simulink model "dobbel_oppdatert_sim"  (R2023b)
settings: Solver=VariableStepAuto  StartTime=0.0  StopTime=inf  FixedStep=0.0001  RelTol=1e-6  AbsTol=1e-6
model workspace (MAT data in the model file):
  SL_ROS_VariableLengthArrays_MaxSizes.CommonInfo.ArrayTruncateAction = 'EmitWarning'
  SL_ROS_VariableLengthArrays_MaxSizes.MsgTypeMap = containers.Map
  SL_ROS_VariableLengthArrays_MaxSizes.MsgTypeMap.serialization.keys = {'std_msgs/Float64MultiArray'}
  SL_ROS_VariableLengthArrays_MaxSizes.MsgTypeMap.serialization.values{1}.PropertyName = 'data'
  SL_ROS_VariableLengthArrays_MaxSizes.MsgTypeMap.serialization.values{1}.DataType = 'double'
  SL_ROS_VariableLengthArrays_MaxSizes.MsgTypeMap.serialization.values{1}.MaxLength = 500
  SL_ROS_VariableLengthArrays_MaxSizes.MsgTypeMap.serialization.uniformity = 0
  SL_ROS_VariableLengthArrays_MaxSizes.MsgTypeMap.serialization.keyType = 'char'
  SL_ROS_VariableLengthArrays_MaxSizes.MsgTypeMap.serialization.valueType = 'any'
values from neighbouring files (symbols this model uses):
  B = 10    [LoneWolfParams.m]
  C = 1.9    [LoneWolfParams.m]
  D = 1    [LoneWolfParams.m]
  g = 9.81    [LoneWolfParams.m]
  Iz = (1/12) * m * (with^2 + len^2)    [LoneWolfParams.m]
  m = 375    [LoneWolfParams.m]
  xdotinit = 1e-3    (= 0.001)    [LoneWolfParams.m]
undefined symbols (not defined in the file or in its folder): latitude, longitude
libraries: ros2lib x11, simulink x2, dspstat3 x1, sldrtlib x1
settings Model: Creator=bakke  LastModifiedBy=lonewolf
settings SolverCC: AutoScaleAbsTol=off  EnableFixedStepZeroCrossing=on  MaxZcBracketingIterations=100
settings OptimizationCC: EnhancedBackFolding=on  PassReuseOutputArgsAs=Individual arguments  ZeroExternalMemoryAtStartup=off  ZeroInternalMemoryAtStartup=off  MaxStackSize=64  OptimizeBlockOrder=speed  DifferentSizesBufferReuse=on  OptimizationCustomize=off  EfficientTunableParamExpr=on
settings DebuggingCC: ParameterTunabilityLossMsg=error
settings HardwareCC: ProdBitPerLong=64  ProdHWDeviceType=Intel->x86-64 (Linux 64)  UseEmbeddedCoderFeatures=off
settings RTWCC: Description=Embedded Coder  SystemTargetFile=ert.tlc  HardwareBoard=Robot Operating System 2 (ROS 2)  TLCOptions="-aInlineSetEventsForThisBaseRateFcn=TLC_FALSE -aSuppressMultiTaskScheduler=TLC_FALSE  -aRateBasedStepFcn=0"  TemplateMakefile=ert_default_tmf  Toolchain=Colcon Tools  TargetLang=C++
settings CodeAppCC: ForceParamTrailComments=on  IgnoreCustomStorageClasses=off  OperatorAnnotations=on  SimulinkDataObjDesc=on  SFDataObjDesc=on  InsertBlockDesc=on
settings ERTTargetCC: CodeInterfacePackaging=C++ class  SupportNonInlinedSFcns=on  RootIOFormat=Structure reference

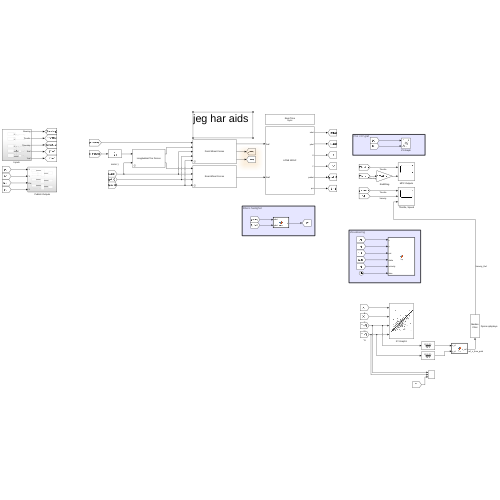
[thumbnail: Simulink's stored preview of the top-level diagram]
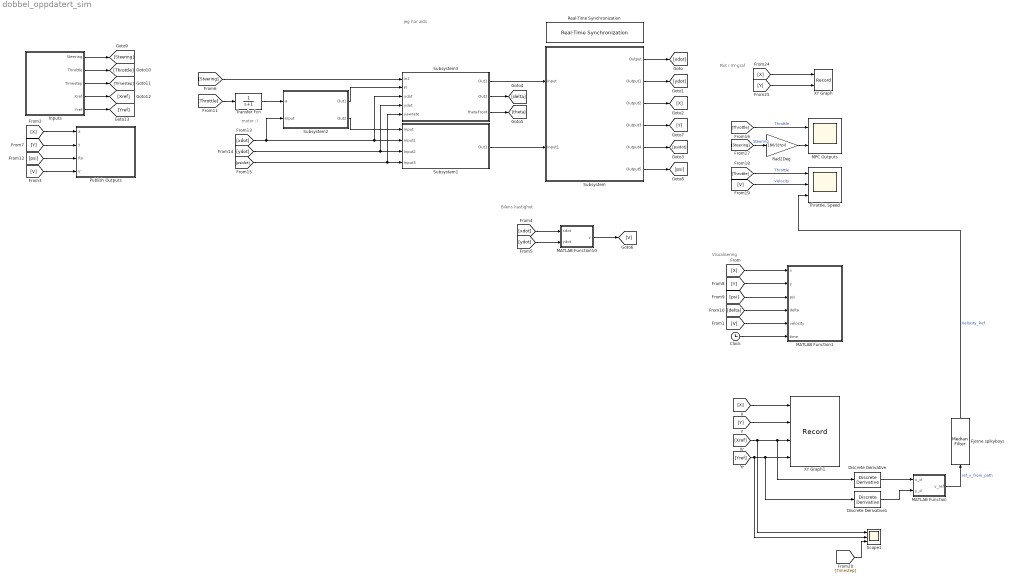
== system dobbel_oppdatert_sim ==
  note: motor :)
  note: jeg har aids
  note: Visualisering
  note: Plot i XY-graf
  note: Bilens hastighet
  Clock : Clock
  Discrete Derivative : simulink/Discrete/Discrete Derivative  gainval=1.0  ICPrevScaledInput=0.0  OutMin=[]  OutMax=[]  OutDataType=fixdt(1, 16)  OutScaling=2^-10  DoSatur=off
  Discrete Derivative1 : simulink/Discrete/Discrete Derivative  gainval=1.0  ICPrevScaledInput=0.0  OutMin=[]  OutMax=[]  OutDataType=fixdt(1, 16)  OutScaling=2^-10  DoSatur=off
  Fjerne spikyboys : dspstat3/Median Filter  WindowLength=5  SimulateUsing=Interpreted execution
      settings: LibrarySourceBlock=|
      | dspfdesign/Median
      | Filter
  Inputs : Subsystem
  MATLAB Function : MATLAB Function  TreatAsAtomicUnit=on
  MATLAB Function1 : MATLAB Function  TreatAsAtomicUnit=on
  MATLAB Function10 : MATLAB Function  TreatAsAtomicUnit=on
  MPC Outputs : Scope  NumInputPorts=2
  Publish Outputs : Subsystem
  Rad2Deg : Gain  Gain=180/(2*pi)
  Real-Time Synchronization : sldrtlib/Real-Time Synchronization  SampleTime=0.1  MaxMissedTicks=1000  ShowMissedTicks=off  YieldWhenWaiting=off
  Scope1 : Scope  NumInputPorts=3
  Subsystem : Subsystem
      mask Display: disp('LONE WOLF');
  Subsystem1 : Subsystem
      mask Display: disp('Rear Wheel Forces');
  Subsystem2 : Subsystem
      mask Display: disp('Longitudinal Tire Forces');
  Subsystem3 : Subsystem
      mask Display: disp('Front Wheel Forces');
  "Throttle, Speed" : Scope  NumInputPorts=3
  Transfer Fcn : TransferFcn  Denominator=[1 1]
  XY Graph : Record  FileSettingsInternal="{\"entries\":[{\"content\":{\"excelSettings\":{\"content\":{},\"type\":\"Streamout.ExcelSettings\"}},\"type\":\"Streamout.FileSettingStorage\",\"uuid\":\"\"}],\"packageUris\":[\"http:\\/\\/schema.mathworks.com\\/mf0\\/streamout_blocks\\/R2020a\"],\"version\":\"1.0\"}"  Layout=[1 1]  SignalsInternal="{\"entries\":[{\"content\":{\"signals\":[{\"content\":{\"blockPath\":[],\"dimensions\":[1],\"domain\":\"\",\"lineColor\":\"#d95319\",\"plots\":[ 1 ],\"port\":1,\"sid\":[\"\"],\"signalID\":1,\"signalName\":\"From24\"},\"type\":\"RecordBlkView.Signal\",\"uuid\":\"\"},{\"content\":{\"blockPath\":[],\"dimensions\":[1],\"domain\":\"\",\"lineColor\":\"#edb120\",\"plots\":[ 1 ],\"port\":2,\"sid\":[\"\"],\"signalID\":2,\"signalName\":\"From25\"},\"type\":\"RecordBlkView.Signal\",\"uuid\":\"\"}]},\"type\":\"RecordBlkView.InputSignals\",\"uuid\":\"\"}],\"packageUris\":[\"http:\\/\\/schema.mathworks.com\\/mf0\\/streamout_blocks\\/R2020a\"],\"version\":\"1.0\"}"  VisualizationBindings="{\"xyplotplugin\":{\"info\":[{\"series\":[{\"bindingParametersList\":[{\"parameter\":\"X-Axis\",\"signalID\":1,\"signalName\":\"From24\"},{\"parameter\":\"Y-Axis\",\"signalID\":2,\"signalName\":\"From25\"}],\"seriesID\":0}],\"subplotID\":1}]}}"  CompatibilityTag=XY
  XY Graph1 : Record  FileSettingsInternal="{\"entries\":[{\"content\":{\"excelSettings\":{\"content\":{},\"type\":\"Streamout.ExcelSettings\"}},\"type\":\"Streamout.FileSettingStorage\",\"uuid\":\"\"}],\"packageUris\":[\"http:\\/\\/schema.mathworks.com\\/mf0\\/streamout_blocks\\/R2020a\"],\"version\":\"1.0\"}"  Layout=[1 1]  SignalsInternal="{\"entries\":[{\"content\":{\"signals\":[{\"content\":{\"blockPath\":[],\"dimensions\":[1],\"domain\":\"\",\"lineColor\":\"#a2142f\",\"plots\":[ 1 ],\"port\":1,\"sid\":[\"\"],\"signalID\":1,\"signalName\":\"X\"},\"type\":\"RecordBlkView.Signal\",\"uuid\":\"\"},{\"content\":{\"blockPath\":[],\"dimensions\":[1],\"domain\":\"\",\"lineColor\":\"#139fff\",\"plots\":[ 1 ],\"port\":2,\"sid\":[\"\"],\"signalID\":2,\"signalName\":\"Y\"},\"type\":\"RecordBlkView.Signal\",\"uuid\":\"\"},{\"content\":{\"blockPath\":[],\"dimensions\":[1],\"domain\":\"\",\"lineColor\":\"#a2142f\",\"plots\":[ 1 ],\"port\":3,\"sid\":[\"\"],\"signalID\":3,\"signalName\":\"Xr\"},\"type\":\"RecordBlkView.Signal\",\"uuid\":\"\"},{\"content\":{\"blockPath\":[],\"dimensions\":[1],\"domain\":\"\",\"lineColor\":\"#139fff\",\"plots\":[ 1 ],\"port\":4,\"sid\":[\"\"],\"signalID\":4,\"signalName\":\"Yr\"},\"type\":\"RecordBlkView.Signal\",\"uuid\":\"\"}]},\"type\":\"RecordBlkView.InputSignals\",\"uuid\":\"\"}],\"packageUris\":[\"http:\\/\\/schema.mathworks.com\\/mf0\\/streamout_blocks\\/R2020a\"],\"version\":\"1.0\"}"  VisualizationBindings="{\"xyplotplugin\":{\"info\":[{\"series\":[{\"bindingParametersList\":[{\"parameter\":\"X-Axis\",\"signalID\":3,\"signalName\":\"Xr\"},{\"parameter\":\"Y-Axis\",\"signalID\":4,\"signalName\":\"Yr\"},{\"parameter\":\"X-Axis\",\"signalID\":3,\"signalName\":\"Xr\"},{\"parameter\":\"Y-Axis\",\"signalID\":4,\"signalName\":\"Yr\"},{\"parameter\":\"X-Axis\",\"signalID\":3,\"signalName\":\"Xr\"},{\"parameter\":\"Y-Axis\",\"signalID\":4,\"signalName\":\"Yr\"}],\"seriesID\":0},{\"bindingParametersList\":[{\"parameter\":\"X-Axis\",\"signalID\":1,\"signalName\":\"X\"},{\"parameter\":\"Y-Axis\",\"signalID\":2,\"signalName\":\"Y\"},{\"parameter\":\"X-Axis\",\"signalID\":1,\"signalName\":\"X\"},{\"parameter\":\"Y-Axis\",\"signalID\":2,\"signalName\":\"Y\"}],\"seriesID\":1}],\"subplotID\":1}]}}"  CompatibilityTag=XY
  wires:
  MATLAB Function10/1(v) -> [V]
  [ydot] -> MATLAB Function10/2(ydot)
  Subsystem/1(Output) -> [xdot]
  [xdot] -> MATLAB Function10/1(xdot)
  Subsystem/2(Output1) -> [ydot]
  Subsystem/5(Output4) -> [psidot]
  Subsystem/4(Output3) -> [Y]
  Subsystem/3(Output2) -> [X]
  Subsystem/6(Output5) -> [psi]
  [Y] -> XY Graph/2
  [X] -> XY Graph/1
  Subsystem1/1(Out1) -> Subsystem/2(Input1)
  Subsystem2/2(Out2) -> Subsystem1/1(Input)
  Subsystem2/1(Out1) -> Subsystem3/2(Fl)
  Subsystem3/1(Out1) -> Subsystem/1(Input)
  [xdot] -> Subsystem2/2(Input), Subsystem3/3(xdot), Subsystem1/2(Input1)
  [ydot] -> Subsystem3/4(ydot), Subsystem1/3(Input2)
  [psidot] -> Subsystem3/5(yawrate), Subsystem1/4(Input3)
  Subsystem3/3(thetaFront) -> [theta]
  Subsystem3/2(Out2) -> [delta]
  [X] -> MATLAB Function1/1(x)
  [Y] -> MATLAB Function1/2(y)
  [psi] -> MATLAB Function1/3(psi)
  [delta] -> MATLAB Function1/4(delta)
  Clock/1 -> MATLAB Function1/6(time)
  Transfer Fcn/1 -> Subsystem2/1(a)
  [X] -> Publish Outputs/1(X)
  [Y] -> Publish Outputs/2(Y)
  [psi] -> Publish Outputs/3(Psi)
  [V] -> Publish Outputs/4(V)
  [V] -> MATLAB Function1/5(velocity)
  Inputs/1(Steering) -> [Steering]
  Inputs/2(Throttle) -> [Throttle]
  [Throttle] -> Transfer Fcn/1
  [Steering] -> Subsystem3/1(In2)
  [Throttle] -> MPC Outputs/1  "Throttle"
  [Steering] -> Rad2Deg/1  "Steering"
  [Throttle] -> "Throttle, Speed"/1  "Throttle"
  [V] -> "Throttle, Speed"/2  "Velocity"
  Rad2Deg/1 -> MPC Outputs/2
  Inputs/3(Timestep) -> [Timestep]
  Inputs/4(Xref) -> [Xref]
  Inputs/5(Yref) -> [Yref]
  [X] -> XY Graph1/1
  [Y] -> XY Graph1/2
  [Xref] -> Scope1/1, Discrete Derivative/1, XY Graph1/3
  [Yref] -> Scope1/2, Discrete Derivative1/1, XY Graph1/4
  Discrete Derivative/1 -> MATLAB Function/1(x_d)
  Discrete Derivative1/1 -> MATLAB Function/2(y_d)
  MATLAB Function/1(v_ref) -> Fjerne spikyboys/1  "ref_v_from_path"
  [Timestep] -> Scope1/3
  Fjerne spikyboys/1 -> "Throttle, Speed"/3  "Velocity_Ref"

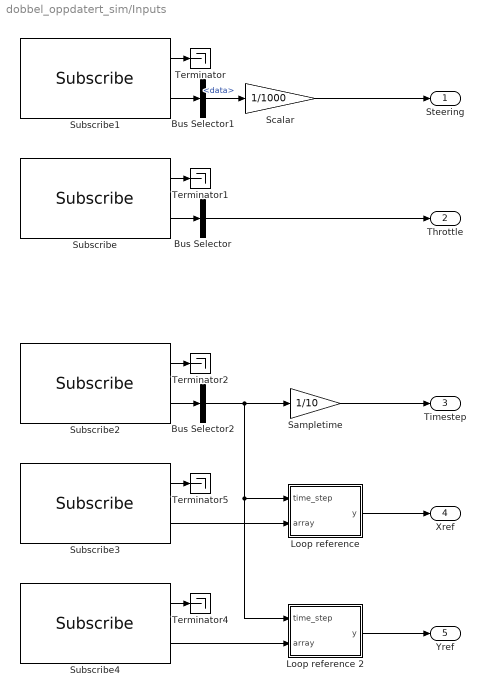
== system dobbel_oppdatert_sim/Inputs ==
  Bus Selector : BusSelector  OutputSignals=data  OutputAsBus=on
  Bus Selector1 : BusSelector  OutputSignals=data
  Bus Selector2 : BusSelector  OutputSignals=data  OutputAsBus=on
  Loop reference : MATLAB Function  TreatAsAtomicUnit=on
  Loop reference 2 : MATLAB Function  TreatAsAtomicUnit=on
  Sampletime : Gain  Gain=1/10
  Scalar : Gain  Gain=1/1000
  Subscribe : ros2lib/Subscribe  topicSource=Specify your own  topic=/lw_portenta_throttle  messageType=std_msgs/Int64  sampleTime=0.1  QOSHistory=Keep last  QOSDepth=1  QOSReliability=Reliable  QOSDurability=Volatile
  Subscribe1 : ros2lib/Subscribe  topicSource=Specify your own  topic=/lw_portenta_steering  messageType=std_msgs/Int64  sampleTime=0.1  QOSHistory=Keep last  QOSDepth=1  QOSReliability=Reliable  QOSDurability=Volatile
  Subscribe2 : ros2lib/Subscribe  topicSource=Specify your own  topic=/timestep  messageType=std_msgs/Int64  sampleTime=0.1  QOSHistory=Keep last  QOSDepth=1  QOSReliability=Reliable  QOSDurability=Volatile
  Subscribe3 : ros2lib/Subscribe  topicSource=Specify your own  topic=/xref  messageType=std_msgs/Float64MultiArray  sampleTime=0.1  QOSHistory=Keep last  QOSDepth=1  QOSReliability=Reliable  QOSDurability=Volatile
  Subscribe4 : ros2lib/Subscribe  topicSource=Specify your own  topic=/yref  messageType=std_msgs/Float64MultiArray  sampleTime=0.1  QOSHistory=Keep last  QOSDepth=1  QOSReliability=Reliable  QOSDurability=Volatile
  Terminator{,1..2,4..5} (5 alike) : Terminator
  Steering : Outport
  Throttle : Outport  Port=2
  Timestep : Outport  Port=3
  Xref : Outport  Port=4
  Yref : Outport  Port=5
  wires:
  Subscribe/1 -> Terminator1/1
  Subscribe1/1 -> Terminator/1
  Subscribe/2 -> Bus Selector/1
  Subscribe1/2 -> Bus Selector1/1
  Bus Selector1/1 -> Scalar/1  "<data>"
  Bus Selector/1 -> Throttle/1
  Scalar/1 -> Steering/1
  Subscribe2/1 -> Terminator2/1
  Subscribe2/2 -> Bus Selector2/1
  Bus Selector2/1 -> Loop reference 2/1(time_step), Loop reference/1(time_step), Sampletime/1
  Sampletime/1 -> Timestep/1
  Subscribe4/1 -> Terminator4/1
  Subscribe4/2 -> Loop reference 2/2(array)
  Subscribe3/2 -> Loop reference/2(array)
  Loop reference/1(y) -> Xref/1
  Loop reference 2/1(y) -> Yref/1
  Subscribe3/1 -> Terminator5/1

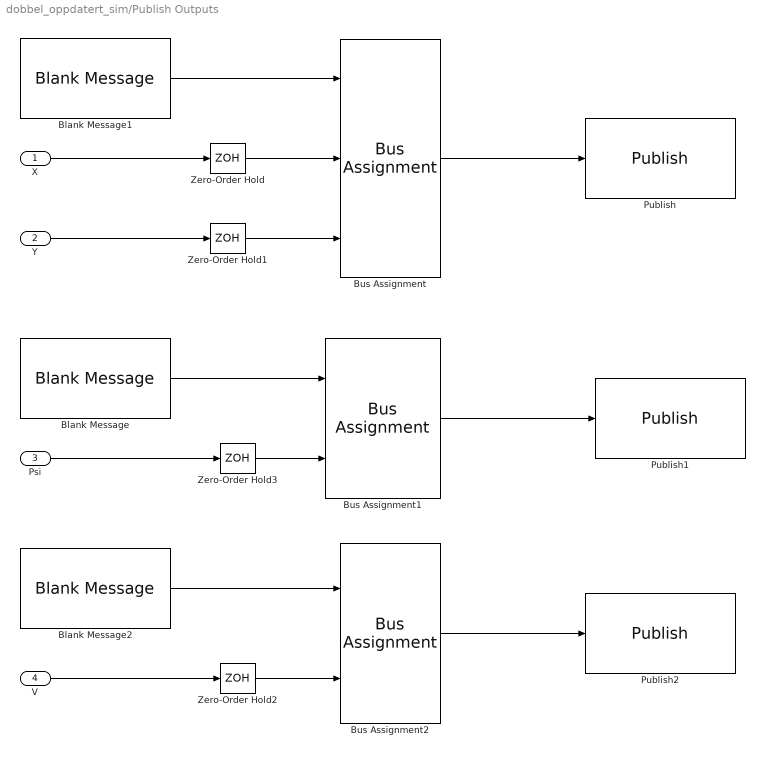
== system dobbel_oppdatert_sim/Publish Outputs ==
  X : Inport
  Y : Inport  Port=2
  Psi : Inport  Port=3
  V : Inport  Port=4
  Blank Message : ros2lib/Blank Message  messageClass=Message  entityType=geometry_msgs/PoseWithCovarianceStamped  messageType=geometry_msgs/PoseWithCovarianceStamped  SampleTime=0.1
  Blank Message1 : ros2lib/Blank Message  messageClass=Message  entityType=sensor_msgs/NavSatFix  messageType=sensor_msgs/NavSatFix  SampleTime=0.1
  Blank Message2 : ros2lib/Blank Message  messageClass=Message  entityType=geometry_msgs/TwistWithCovarianceStamped  messageType=geometry_msgs/TwistWithCovarianceStamped  SampleTime=0.1
  Bus Assignment : BusAssignment  AssignedSignals=latitude,longitude
  Bus Assignment1 : BusAssignment  AssignedSignals=pose.pose.position.z
  Bus Assignment2 : BusAssignment  AssignedSignals=twist.twist.linear.x
  Publish : ros2lib/Publish  topicSource=Specify your own  topic=/vectornav/gnss  messageType=sensor_msgs/NavSatFix  QOSHistory=Keep last  QOSDepth=1  QOSReliability=Reliable  QOSDurability=Volatile
  Publish1 : ros2lib/Publish  topicSource=Specify your own  topic=/vectornav/pose  messageType=geometry_msgs/PoseWithCovarianceStamped  QOSHistory=Keep last  QOSDepth=1  QOSReliability=Reliable  QOSDurability=Volatile
  Publish2 : ros2lib/Publish  topicSource=Specify your own  topic=/vectornav/velocity_body  messageType=geometry_msgs/TwistWithCovarianceStamped  QOSHistory=Keep last  QOSDepth=1  QOSReliability=Reliable  QOSDurability=Volatile
  Zero-Order Hold{,1..3} (4 alike) : ZeroOrderHold  SampleTime=0.1
  wires:
  Blank Message/1 -> Bus Assignment1/1
  Bus Assignment1/1 -> Publish1/1
  Zero-Order Hold2/1 -> Bus Assignment2/2
  Bus Assignment2/1 -> Publish2/1
  Zero-Order Hold3/1 -> Bus Assignment1/2
  Psi/1 -> Zero-Order Hold3/1
  Blank Message1/1 -> Bus Assignment/1
  V/1 -> Zero-Order Hold2/1
  X/1 -> Zero-Order Hold/1
  Zero-Order Hold/1 -> Bus Assignment/2
  Bus Assignment/1 -> Publish/1
  Blank Message2/1 -> Bus Assignment2/1
  Y/1 -> Zero-Order Hold1/1
  Zero-Order Hold1/1 -> Bus Assignment/3

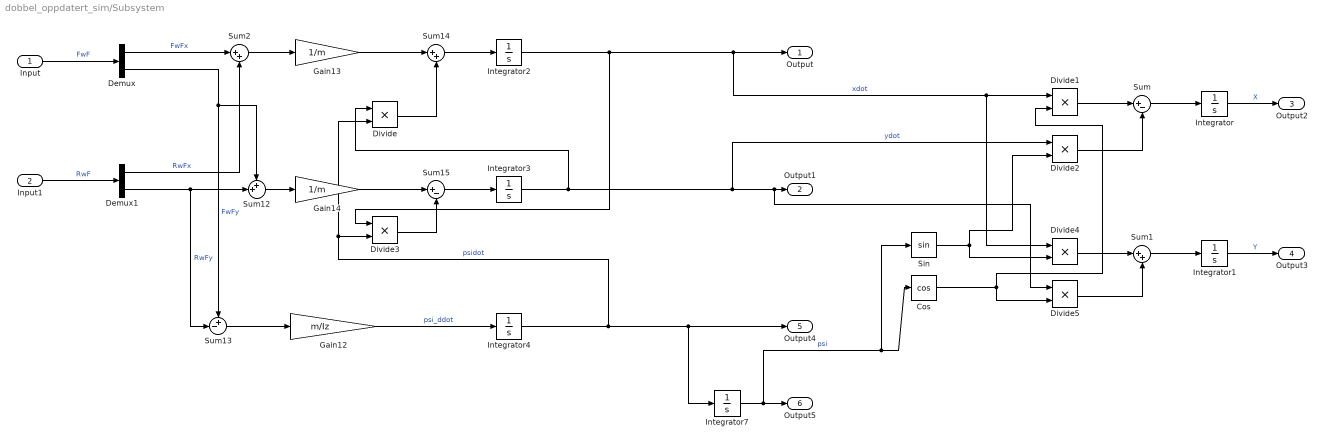
== system dobbel_oppdatert_sim/Subsystem ==
  Input : Inport
  Input1 : Inport  Port=2
  Cos : Trigonometry  Operator=cos
  Demux : Demux  Outputs=2
  Demux1 : Demux  Outputs=2
  Divide{,1..5} (6 alike) : Product  Inputs=**
  Gain12 : Gain  Gain=m/Iz
  Gain13 : Gain  Gain=1/m
  Gain14 : Gain  Gain=1/m
  Integrator{,1,3..4,7} (5 alike) : Integrator
  Integrator2 : Integrator  InitialCondition=xdotinit
  Sin : Trigonometry
  Sum : Sum  Inputs=|+-
  Sum1 : Sum  Inputs=|++
  Sum12 : Sum  Inputs=++|
  Sum13 : Sum  Inputs=+-|
  Sum14 : Sum  Inputs=|++
  Sum15 : Sum  Inputs=|+-
  Sum2 : Sum  Inputs=|++
  Output : Outport
  Output1 : Outport  Port=2
  Output2 : Outport  Port=3
  Output3 : Outport  Port=4
  Output4 : Outport  Port=5
  Output5 : Outport  Port=6
  wires:
  Demux1/1 -> Sum2/2  "RwFx"
  Input/1 -> Demux/1  "FwF"
  Demux/1 -> Sum2/1  "FwFx"
  Demux1/2 -> Sum12/2, Sum13/2  "RwFy"
  Integrator2/1 -> Divide1/1, Divide4/1, Output/1, Divide3/1  "xdot"
  Sum13/1 -> Gain12/1
  Integrator4/1 -> Output4/1, Integrator7/1, Divide3/2, Divide/2  "psidot"
  Sum14/1 -> Integrator2/1
  Demux/2 -> Sum12/1, Sum13/1  "FwFy"
  Input1/1 -> Demux1/1  "RwF"
  Gain13/1 -> Sum14/1
  Integrator7/1 -> Output5/1, Cos/1, Sin/1  "psi"
  Gain14/1 -> Sum15/1
  Integrator3/1 -> Divide5/1, Output1/1, Divide2/1, Divide/1  "ydot"
  Divide3/1 -> Sum15/2
  Gain12/1 -> Integrator4/1  "psi_ddot"
  Sum2/1 -> Gain13/1
  Sum15/1 -> Integrator3/1
  Sum12/1 -> Gain14/1
  Divide/1 -> Sum14/2
  Cos/1 -> Divide5/2, Divide1/2
  Sin/1 -> Divide4/2, Divide2/2
  Divide1/1 -> Sum/1
  Divide2/1 -> Sum/2
  Divide4/1 -> Sum1/1
  Divide5/1 -> Sum1/2
  Sum/1 -> Integrator/1
  Integrator/1 -> Output2/1  "X"
  Sum1/1 -> Integrator1/1
  Integrator1/1 -> Output3/1  "Y"

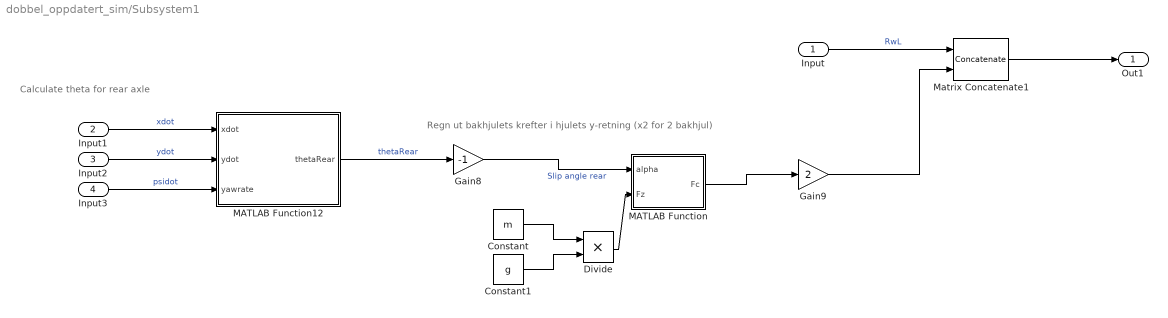
== system dobbel_oppdatert_sim/Subsystem1 ==
  note: Regn ut bakhjulets krefter i hjulets y-retning (x2 for 2 bakhjul)
  note: Calculate theta for rear axle
  Input : Inport
  Input1 : Inport  Port=2
  Input2 : Inport  Port=3
  Input3 : Inport  Port=4
  Constant : Constant  Value=m
  Constant1 : Constant  Value=g
  Divide : Product  Inputs=**
  Gain8 : Gain  Gain=-1
  Gain9 : Gain  Gain=2
  MATLAB Function : MATLAB Function  TreatAsAtomicUnit=on
  MATLAB Function12 : MATLAB Function  TreatAsAtomicUnit=on
  Matrix Concatenate1 : Concatenate  Mode=Multidimensional array
  Out1 : Outport
  wires:
  Matrix Concatenate1/1 -> Out1/1
  Gain8/1 -> MATLAB Function/1(alpha)  "Slip angle rear"
  MATLAB Function12/1(thetaRear) -> Gain8/1  "thetaRear"
  Gain9/1 -> Matrix Concatenate1/2
  Input/1 -> Matrix Concatenate1/1  "RwL"
  Input3/1 -> MATLAB Function12/3(yawrate)  "psidot"
  Input2/1 -> MATLAB Function12/2(ydot)  "ydot"
  Input1/1 -> MATLAB Function12/1(xdot)  "xdot"
  Constant1/1 -> Divide/2
  Constant/1 -> Divide/1
  Divide/1 -> MATLAB Function/2(Fz)
  MATLAB Function/1(Fc) -> Gain9/1

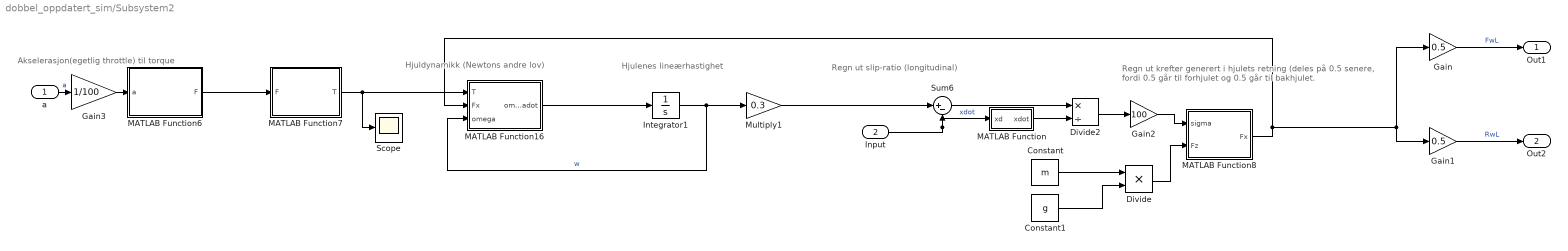
== system dobbel_oppdatert_sim/Subsystem2 ==
  note: Akselerasjon(egetlig throttle) til torque
  note: Hjulenes lineærhastighet
  note: Regn ut krefter generert i hjulets retning (deles på 0.5 senere, fordi 0.5 går til forhjulet og 0.5 går til bakhjulet.
  note: Regn ut slip-ratio (longitudinal)
  note: Hjuldynamikk (Newtons andre lov)
  a : Inport
  Input : Inport  Port=2
  Constant : Constant  Value=m
  Constant1 : Constant  Value=g
  Divide : Product  Inputs=**
  Divide2 : Product  Inputs=*/
  Gain : Gain  Gain=0.5
  Gain1 : Gain  Gain=0.5
  Gain2 : Gain  Gain=100
  Gain3 : Gain  Gain=1/100
  Integrator1 : Integrator  InitialCondition=(xdotinit)/0.3
  MATLAB Function : MATLAB Function  TreatAsAtomicUnit=on
  MATLAB Function16 : MATLAB Function  TreatAsAtomicUnit=on
  MATLAB Function6 : MATLAB Function  TreatAsAtomicUnit=on
  MATLAB Function7 : MATLAB Function  TreatAsAtomicUnit=on
  MATLAB Function8 : MATLAB Function  TreatAsAtomicUnit=on
  Multiply1 : Gain  Gain=0.3
  Scope : Scope
  Sum6 : Sum  Inputs=|+-
  Out1 : Outport
  Out2 : Outport  Port=2
  wires:
  Constant1/1 -> Divide/2
  MATLAB Function8/1(Fx) -> MATLAB Function16/2(Fx), Gain1/1, Gain/1
  Divide2/1 -> Gain2/1
  MATLAB Function7/1(T) -> Scope/1, MATLAB Function16/1(T)
  MATLAB Function16/1(omegadot) -> Integrator1/1
  MATLAB Function6/1(F) -> MATLAB Function7/1(F)
  Integrator1/1 -> MATLAB Function16/3(omega), Multiply1/1  "w"
  Multiply1/1 -> Sum6/1
  Constant/1 -> Divide/1
  Divide/1 -> MATLAB Function8/2(Fz)
  Sum6/1 -> Divide2/1
  Gain1/1 -> Out2/1  "RwL"
  Gain/1 -> Out1/1  "FwL"
  a/1 -> Gain3/1  "a"
  Input/1 -> MATLAB Function/1(xd), Sum6/2  "xdot"
  MATLAB Function/1(xdot) -> Divide2/2
  Gain2/1 -> MATLAB Function8/1(sigma)
  Gain3/1 -> MATLAB Function6/1(a)

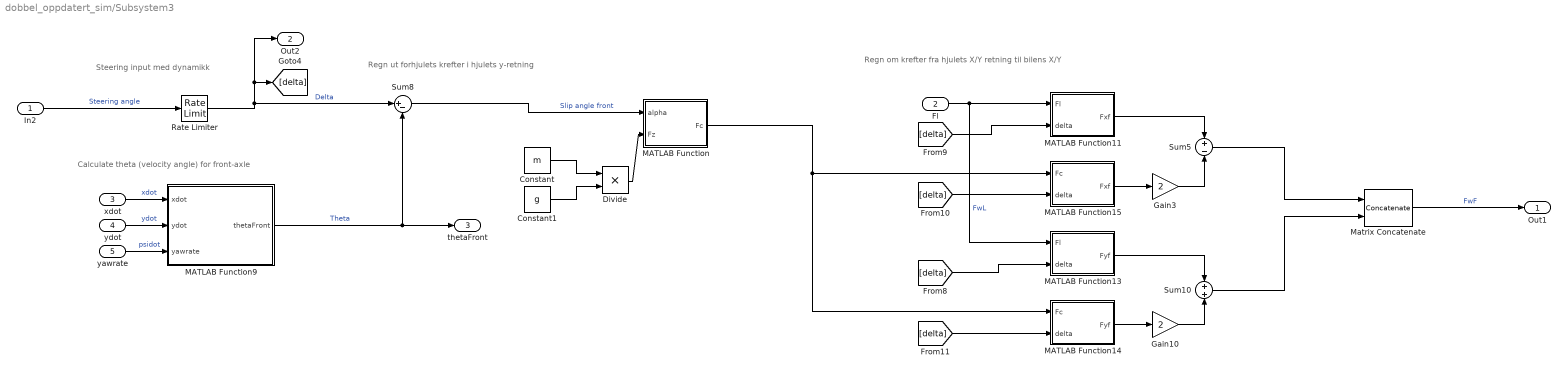
== system dobbel_oppdatert_sim/Subsystem3 ==
  note: Regn om krefter fra hjulets X/Y retning til bilens X/Y
  note: Steering input med dynamikk
  note: Regn ut forhjulets krefter i hjulets y-retning
  note: Calculate theta (velocity angle) for front-axle
  In2 : Inport
  Fl : Inport  Port=2
  xdot : Inport  Port=3
  ydot : Inport  Port=4
  yawrate : Inport  Port=5
  Constant : Constant  Value=m
  Constant1 : Constant  Value=g
  Divide : Product  Inputs=**
  Gain10 : Gain  Gain=2
  Gain3 : Gain  Gain=2
  MATLAB Function : MATLAB Function  TreatAsAtomicUnit=on
  MATLAB Function11 : MATLAB Function  TreatAsAtomicUnit=on
  MATLAB Function13 : MATLAB Function  TreatAsAtomicUnit=on
  MATLAB Function14 : MATLAB Function  TreatAsAtomicUnit=on
  MATLAB Function15 : MATLAB Function  TreatAsAtomicUnit=on
  MATLAB Function9 : MATLAB Function  TreatAsAtomicUnit=on
  Matrix Concatenate : Concatenate  Mode=Multidimensional array
  Rate Limiter : RateLimiter  RisingSlewLimit=pi/2  FallingSlewLimit=-pi/2
  Sum10 : Sum  Inputs=+|+
  Sum5 : Sum  Inputs=+|-
  Sum8 : Sum  Inputs=|+-
  Out1 : Outport
  Out2 : Outport  Port=2
  thetaFront : Outport  Port=3
  wires:
  Gain3/1 -> Sum5/2
  Sum10/1 -> Matrix Concatenate/2
  MATLAB Function11/1(Fxf) -> Sum5/1
  [delta] -> MATLAB Function11/2(delta)
  MATLAB Function15/1(Fxf) -> Gain3/1
  Sum5/1 -> Matrix Concatenate/1
  [delta] -> MATLAB Function15/2(delta)
  MATLAB Function9/1(thetaFront) -> Sum8/2, thetaFront/1  "Theta"
  Gain10/1 -> Sum10/2
  [delta] -> MATLAB Function14/2(delta)
  MATLAB Function13/1(Fyf) -> Sum10/1
  Sum8/1 -> MATLAB Function/1(alpha)  "Slip angle front"
  MATLAB Function14/1(Fyf) -> Gain10/1
  [delta] -> MATLAB Function13/2(delta)
  Rate Limiter/1 -> [delta], Out2/1, Sum8/1  "Delta"
  Matrix Concatenate/1 -> Out1/1  "FwF"
  In2/1 -> Rate Limiter/1  "Steering angle"
  Fl/1 -> MATLAB Function11/1(Fl), MATLAB Function13/1(Fl)  "FwL"
  xdot/1 -> MATLAB Function9/1(xdot)  "xdot"
  ydot/1 -> MATLAB Function9/2(ydot)  "ydot"
  yawrate/1 -> MATLAB Function9/3(yawrate)  "psidot"
  Constant/1 -> Divide/1
  Constant1/1 -> Divide/2
  Divide/1 -> MATLAB Function/2(Fz)
  MATLAB Function/1(Fc) -> MATLAB Function15/1(Fc), MATLAB Function14/1(Fc)

== matlab function dobbel_oppdatert_sim/Subsystem2/MATLAB Function8 ==
  data: sigma input; Fz input; Fx output; B parameter; C parameter; D parameter; E parameter
function Fx = fcn(sigma, Fz, B, C, D, E)

mu = D*sin(C*atan(B*sigma-E*(B*sigma-atan(B*sigma))));

Fx = mu * Fz;

== matlab function dobbel_oppdatert_sim/Subsystem3/MATLAB Function9 ==
  data: xdot input; thetaFront output; ydot input; yawrate input
function thetaFront = fcn(xdot, ydot, yawrate)

thetaFront = atan((ydot+yawrate*1.4)/xdot);

== matlab function dobbel_oppdatert_sim/Subsystem1/MATLAB Function12 ==
  data: xdot input; thetaRear output; ydot input; yawrate input
function thetaRear = fcn(xdot, ydot, yawrate)

thetaRear = atan((ydot-yawrate*1.6)/xdot);

== matlab function dobbel_oppdatert_sim/Subsystem3/MATLAB Function13 ==
  data: Fl input; Fyf output; delta input
function Fyf = fcn(Fl, delta)

Fyf = Fl*sin(delta);

== matlab function dobbel_oppdatert_sim/Subsystem3/MATLAB Function14 ==
  data: Fc input; delta input; Fyf output
function Fyf = fcn(Fc, delta)

Fyf = Fc*cos(delta);

== matlab function dobbel_oppdatert_sim/Subsystem3/MATLAB Function15 ==
  data: Fc input; Fxf output; delta input
function Fxf = fcn(Fc, delta)

Fxf = Fc*sin(delta);

== matlab function dobbel_oppdatert_sim/Subsystem2/MATLAB Function16 ==
  data: T input; omegadot output; Fx input; omega input
function omegadot = fcn(T, Fx, omega)

omegadot = (T - 0.3 * Fx - 11 * omega)/0.5;

% 0.5 = Hjulets treghetsmoment

== matlab function dobbel_oppdatert_sim/MATLAB Function1 ==
  settings: updateMethod=DISCRETE  sampleTime=0.1
  data: x input; y input; psi input; delta input; velocity input; time input
function fnc(x, y, psi, delta, velocity, time)
    persistent xmin xmax ymin ymax vehiclePathX vehiclePathY vehicleFig pathPlot leftWheelPatch rightWheelPatch rearLeftWheelPatch rearRightWheelPatch lwPatch velocityPlot deltaPlot timeArray deltaArray velocityArray
    
    lwWidth = 2.4;
    lwHeight = 1.2;
    wheelWidth = 0.66;
    wheelHeight = 0.22;

    if isempty(vehicleFig)
        vehicleFig = figure('WindowState','maximized');
        hold on;
        subplot(3,6,[1:3 7:9 13:15]);
        pathPlot = plot(NaN, NaN, 'k-', 'LineWidth', 2);
        axis equal;
        grid on;
        title('Lone Wolf Simulator')
        xlabel('X-position')
        ylabel('Y-position')
        leftWheelPatch = patch('XData', [], 'YData', [], 'FaceColor', 'k', 'EdgeColor', 'k');
        rightWheelPatch = patch('XData', [], 'YData', [], 'FaceColor', 'k', 'EdgeColor', 'k');
        rearLeftWheelPatch = patch('XData', [], 'YData', [], 'FaceColor', 'k', 'EdgeColor', 'k');
        rearRightWheelPatch = patch('XData', [], 'YData', [], 'FaceColor', 'k', 'EdgeColor', 'k');
        lwPatch = patch('XData', [], 'YData', [], 'FaceColor', 'r', 'EdgeColor', 'k');
        xmin = -15;
        xmax = 15;
        ymin = -15;
        ymax = 15;

        timeArray = [];
        velocityArray = [];
        deltaArray = [];

        subplot(3,6,4:6);
        velocityPlot = plot(NaN, NaN, 'g-', 'LineWidth', 2);
        ylabel('Velocity (km/h)')
        ylim([-5, 80])
        grid on;
        subplot(3,6,10:12);
        deltaPlot = plot(NaN, NaN, 'b-', 'LineWidth', 2);
        ylabel('Steering angle (rad)')
        ylim([-1, 1])
        grid on;
        subplot(3,6,16:18);
        latErrorPlot = plot(NaN, NaN, 'k-', 'LineWidth', 2);
        ylabel('Lateral error (m)')
        ylim([-1, 1])
        grid on;
    end

    if isempty(vehiclePathX)
        vehiclePathX = [];
    end
    
    if isempty(vehiclePathY)
        vehiclePathY = [];
    end
    
    subplot(3,6,[1:3 7:9 13:15]);
    vehiclePathX(end+1) = x;
    vehiclePathY(end+1) = y;
    timeArray(end+1) = time;
    deltaArray(end+1) = delta;
    velocityArray(end+1) = velocity*3.6;

    leftWheelVertices = [-wheelWidth/2, -wheelHeight/2;
                    wheelWidth/2, -wheelHeight/2;
                    wheelWidth/2, wheelHeight/2;
                    -wheelWidth/2, wheelHeight/2];

    rightWheelVertices = [-wheelWidth/2, -wheelHeight/2;
                    wheelWidth/2, -wheelHeight/2;
                    wheelWidth/2, wheelHeight/2;
                    -wheelWidth/2, wheelHeight/2];

    rearLeftWheelVertices = [-wheelWidth/2, -wheelHeight/2;
                    wheelWidth/2, -wheelHeight/2;
                    wheelWidth/2, wheelHeight/2;
                    -wheelWidth/2, wheelHeight/2];

    rearRightWheelVertices = [-wheelWidth/2, -wheelHeight/2;
                    wheelWidth/2, -wheelHeight/2;
                    wheelWidth/2, wheelHeight/2;
                    -wheelWidth/2, wheelHeight/2];

    lwVertices = [-lwWidth/2, -lwHeight/2;
                    lwWidth/2, -lwHeight/2;
                    lwWidth/2, lwHeight/2;
                    -lwWidth/2, lwHeight/2];
    
    R = [cos(psi), -sin(psi); sin(psi), cos(psi)];
    rotatedLW = (R * lwVertices')';
    fW = [cos(psi+delta), -sin(psi+delta); sin(psi+delta), cos(psi+delta)];
    rW = [cos(psi), -sin(psi); sin(psi), cos(psi)];
    rotatedLeftWheel = (fW * leftWheelVertices')';
    rotatedRightWheel = (fW * rightWheelVertices')';
    rotatedRearLeftWheel = (rW * rearLeftWheelVertices')';
    rotatedRearRightWheel = (rW * rearRightWheelVertices')';
    
    translatedLW = rotatedLW + [x, y];
    translatedLeftWheel = rotatedLeftWheel + [x + cos(psi + pi/2) + cos(psi), y + sin(psi + pi/2) + sin(psi)];
    translatedRightWheel = rotatedRightWheel + [x + cos(psi - pi/2) + cos(psi), y + sin(psi - pi/2) + sin(psi)];
    translatedRearLeftWheel = rotatedRearLeftWheel + [x + cos(psi + pi/2) - cos(psi), y + sin(psi + pi/2) - sin(psi)];
    translatedRearRightWheel = rotatedRearRightWheel + [x + cos(psi - pi/2) - cos(psi), y + sin(psi - pi/2) - sin(psi)];
    
    set(leftWheelPatch, 'XData', translatedLeftWheel(:,1), 'YData', translatedLeftWheel(:,2));
    set(rightWheelPatch, 'XData', translatedRightWheel(:,1), 'YData', translatedRightWheel(:,2));
    set(rearLeftWheelPatch, 'XData', translatedRearLeftWheel(:,1), 'YData', translatedRearLeftWheel(:,2));
    set(rearRightWheelPatch, 'XData', translatedRearRightWheel(:,1), 'YData', translatedRearRightWheel(:,2));
    set(lwPatch, 'XData', translatedLW(:,1), 'YData', translatedLW(:,2));
    set(pathPlot, 'XData', vehiclePathX, 'YData', vehiclePathY);

    
    xlim([x-30, x+30]);
    if x - 15 < xmin
        xmin = x-15;
    end
    if x + 15 > xmax
        xmax = x+15;
    end
    ylim([y-30, y+30]);
    if y - 15 < ymin
        ymin = y-15;
    end
    if y + 15 > ymax
        ymax = y+15;
    end
    subplot(3,6,4:6);
    xlim([time-10, time+2]);
    set(velocityPlot, 'XData', timeArray,'YData', velocityArray);

    subplot(3,6,10:12);
    xlim([time-10, time+2]);
    set(deltaPlot, 'XData', timeArray, 'YData', deltaArray);

    drawnow
end

== matlab function dobbel_oppdatert_sim/MATLAB Function ==
  data: x_d input; v_ref output; y_d input
function v_ref = fcn(x_d,y_d)

v_ref = sqrt(x_d^2 + y_d^2);

== matlab function dobbel_oppdatert_sim/Subsystem3/MATLAB Function ==
  data: alpha input; Fc output; Fz input; B parameter; C parameter; D parameter; E parameter
function Fc = fcn(alpha, Fz, B, C, D, E)

mu = D*sin(C*atan(B*alpha-E*(B*alpha-atan(B*alpha))));

Fc = mu * Fz;

== matlab function dobbel_oppdatert_sim/Subsystem2/MATLAB Function ==
  data: xd input; xdot output
function xdot = fcn(xd)

if xd == 0
    xdot = 0.001;
else
    xdot = xd;
end

== matlab function dobbel_oppdatert_sim/Subsystem1/MATLAB Function ==
  data: alpha input; Fc output; Fz input; B parameter; C parameter; D parameter; E parameter
function Fc = fcn(alpha, Fz, B, C, D, E)
mu = D*sin(C*atan(B*alpha-E*(B*alpha-atan(B*alpha))));

Fc = mu * Fz;

== matlab function dobbel_oppdatert_sim/Inputs/Loop reference 2 ==
  data: time_step input; array input; y output
function y = fcn(time_step, array)
    % index = mod(time_step, N_STEPS_REFERENCE) + 1;
    index = mod(time_step, 500) + 1; 
    y = array.data(index);
end

== matlab function dobbel_oppdatert_sim/Inputs/Loop reference ==
  data: time_step input; array input; y output
function y = fcn(time_step, array)
    % index = mod(time_step, N_STEPS_REFERENCE) + 1;
    index = mod(time_step, 500) + 1; 
    y = array.data(index);
end

== matlab function dobbel_oppdatert_sim/MATLAB Function10 ==
  data: xdot input; v output; ydot input
function v = fcn(xdot, ydot)

v = sqrt(xdot^2+ydot^2);

== matlab function dobbel_oppdatert_sim/Subsystem3/MATLAB Function11 ==
  data: Fl input; Fxf output; delta input
function Fxf = fcn(Fl, delta)

Fxf = Fl*cos(delta);

== matlab function dobbel_oppdatert_sim/Subsystem2/MATLAB Function6 ==
  data: a input; F output
function F = fcn(a)

F = 2000*a; % burde være 375 m også må modellen retunes

== matlab function dobbel_oppdatert_sim/Subsystem2/MATLAB Function7 ==
  data: F input; T output
function T = fcn(F)

T = 0.3*F;
